simulink library "EngineSystemSubmodel"  (R2014b)
settings: Solver=ode45  StartTime=0.0  StopTime=10.0  FixedStep=1e-4  RelTol=1e-3
values from neighbouring files (symbols this model uses):
  D_turb_wheel = TC.TC_map.turb.D_wheel    [init_MVM.m]
  delta = 2    [Init8RTFLEX68D.m]    (also in Untitled2.m = fcn(p); fcn.m = zeros(size(p)))
  eta_turb_max = TC.TC_map.turb.eff_max    [init_MVM.m]
  flow_coeff_turb = [-1.585326540339;-4.823836967181;1.5853156139822]    [Init8RTFLEX68D.m]    (also in init_MVM.m = TC.TC_map.turb.flow_fit_coeff)
  fs = 0.0683    [Init8RTFLEX68D.m]    (also in NOxProcessGUI.m = varargin{2}; initHybrid.m; initMV.m; init_MVM.m = 0.0682925799315)
  genset = generators(1)    [runTempCyl4S.m]
  J_tc = TC.SAE_map_comp.inertia    [init_MVM.m]
  kai = 1.7    [Init8RTFLEX68D.m]
  Kb = 1*ones(engines,1)    [initHybrid.m]    (also in initMV.m; init_MVM.m = 1; init_ele.m = 1)
  Kd = 20*ones(engines,1)    [initHybrid.m]    (also in initMV.m; init_MVM.m = 10; init_ele.m = 20)
  Ki = 20*ones(engines,1)    [initHybrid.m]    (also in initMV.m; init_MVM.m = 10; init_ele.m = 20)
  Kp = 20*ones(engines,1)    [initHybrid.m]    (also in initMV.m; init_MVM.m = 10; init_ele.m = 20)
  Load_amp = x(4) + xRef(i)    [GetErrGensetResp.m]    (also in runsimulation.m = 0.55; runsimulationRecovery.m = InitialLoad(jj) + LoadStep(ii))
  Load_bias = x(4)    [GetErrGensetResp.m]    (also in runsimulation.m = 0.15; runsimulationRecovery.m = InitialLoad(jj))
  Load_index = 1    [GetErrGensetResp.m]    (also in runsimulation.m; runsimulationRecovery.m)
  N = x*noMol    [NOxProcessGUI.m]    (also in initHybrid.m = .1*ones(engines,1); initMV.m = .1*ones(engines,1); init_ele.m = 0.1)
  omegat0 = RPM_TC_initial/30*pi    [init_MVM.m]
  Start_time = 50    [GetErrGensetResp.m]    (also in runsimulation.m; runsimulationRecovery.m)
  T_load = 1    [GetErrGensetResp.m]    (also in runsimulation.m; runsimulationRecovery.m)
  T_ref_turb = TC.TC_map.turb.T_ref    [init_MVM.m]
  u0 = 0.2    [init_MVM.m]
  Uc_opt = TC.TC_map.turb.Uc_opt    [init_MVM.m]
  uMax = 1.5*ones(engines,1)    [initHybrid.m]    (also in initMV.m; init_MVM.m = 1.1; init_ele.m = 1.1)
  uMin = 0*ones(engines,1)    [initHybrid.m]    (also in initMV.m; init_MVM.m = 0.1; init_ele.m = 0.1)
undefined symbols (not defined in the file or in its folder): CAIPO, control, CV, cyl, eng, engSCont, omega0, rhoG0, Td, Ti, turbo, u_max, volDisp, vSCont, vSDes
undefined symbols (not defined in the file): comp_eff_map, comp_flow_map, n288_rep, npr, nsp, pr_rep, vComp
libraries: EngineSystemSubmodel x167, simulink x2
(part 3 of 5)

== system EngineSystemSubmodel/Components/EngineCylinderBlock2StrokeBusSSTune ==
  note: `
  note: `
  note: `
  note: `
  note: `
  note: `
  note: `
  uGov : Inport
  phiInj : Inport  Port=2
  cAStartNom : Inport  Port=3
  dCALiftUp : Inport  Port=4
  pTFScav : Inport  Port=5
  pTFExh : Inport  Port=6
  omega : Inport  Port=7
  tempWall : Inport  Port=8
  Bus Creator : BusCreator  Inputs=8
  Bus Creator{1..7} (7 alike) : BusCreator  Inputs=10
  Bus Selector{1..7} (7 alike) : BusSelector  OutputSignals=uGov,phiInj,CAStartNom,EVC,pTFScav,pTFExh,omegaE,tempWall
  Bus Selector{8..11,13..15} (7 alike) : BusSelector  OutputSignals=dmEmb_u,dmEmb_d,Tq,dmb
  Bus Selector16 : BusSelector  OutputSignals=pCyl,phi,V
  EngCylinder2StrokeBusSSTune1 : EngineSystemSubmodel/Components/EngCylinder2StrokeBusSSTune  cylPar=eng.cyl  cylNo=1  cyl=eng.cyl
  EngCylinder2StrokeBusSSTune2 : EngineSystemSubmodel/Components/EngCylinder2StrokeBusSSTune  cylPar=eng.cyl  cylNo=2  cyl=eng.cyl
  EngCylinder2StrokeBusSSTune3 : EngineSystemSubmodel/Components/EngCylinder2StrokeBusSSTune  cylPar=eng.cyl  cylNo=3  cyl=eng.cyl
  EngCylinder2StrokeBusSSTune4 : EngineSystemSubmodel/Components/EngCylinder2StrokeBusSSTune  cylPar=eng.cyl  cylNo=4  cyl=eng.cyl
  EngCylinder2StrokeBusSSTune5 : EngineSystemSubmodel/Components/EngCylinder2StrokeBusSSTune  cylPar=eng.cyl  cylNo=5  cyl=eng.cyl
  EngCylinder2StrokeBusSSTune6 : EngineSystemSubmodel/Components/EngCylinder2StrokeBusSSTune  cylPar=eng.cyl  cylNo=6  cyl=eng.cyl
  EngCylinder2StrokeBusSSTune7 : EngineSystemSubmodel/Components/EngCylinder2StrokeBusSSTune  cylPar=eng.cyl  cylNo=7  cyl=eng.cyl
  Sum{,1..3} (4 alike) : Sum  Inputs=+++++++
  Terminator : Terminator
  pMaxFinder : EngineSystemSubmodel/EngineOperatingParameterCalculation/pMaxFinder
  dmEmbScvg : Outport
  dmEmbExh : Outport  Port=2
  Tq : Outport  Port=3
  pMax : Outport  Port=4
  pCyl1 : Outport  Port=5
  vCyl1 : Outport  Port=6
  dmf : Outport  Port=7
  wires:
  EngCylinder2StrokeBusSSTune1/9 -> Bus Creator1/9
  [toCylinder] -> Bus Selector1/1
  pMaxFinder/1 -> pMax/1  "pMax"
  pMaxFinder/2 -> Terminator/1
  uGov/1 -> Bus Creator/1  "uGov"
  phiInj/1 -> Bus Creator/2  "phiInj"
  cAStartNom/1 -> Bus Creator/3  "CAStartNom"
  dCALiftUp/1 -> Bus Creator/4  "EVC"
  pTFScav/1 -> Bus Creator/5  "pTFScav"
  pTFExh/1 -> Bus Creator/6  "pTFExh"
  omega/1 -> Bus Creator/7  "omegaE"
  Bus Creator/1 -> [toCylinder]
  EngCylinder2StrokeBusSSTune1/1 -> pCyl1/1, Bus Creator1/1  "pCyl"
  EngCylinder2StrokeBusSSTune1/2 -> Bus Creator1/2  "phi"
  EngCylinder2StrokeBusSSTune1/3 -> Bus Creator1/3  "phiIg"
  EngCylinder2StrokeBusSSTune1/4 -> Bus Creator1/4  "dQ"
  EngCylinder2StrokeBusSSTune1/5 -> Bus Creator1/5  "dmEmb_u"
  EngCylinder2StrokeBusSSTune1/6 -> Bus Creator1/6  "dmEmb_d"
  EngCylinder2StrokeBusSSTune1/7 -> Bus Creator1/7  "Tq"
  EngCylinder2StrokeBusSSTune1/8 -> Bus Creator1/8  "dmb"
  Bus Creator1/1 -> Bus Selector16/1, Bus Selector8/1
  Bus Selector8/1 -> Sum/1  "<dmEmb_u>"
  Bus Selector9/1 -> Sum/2  "<dmEmb_u>"
  Bus Selector10/1 -> Sum/3  "<dmEmb_u>"
  Bus Selector11/1 -> Sum/4  "<dmEmb_u>"
  Bus Selector15/1 -> Sum/5  "<dmEmb_u>"
  Bus Selector14/1 -> Sum/6  "<dmEmb_u>"
  Bus Selector13/1 -> Sum/7  "<dmEmb_u>"
  Sum/1 -> dmEmbScvg/1
  Bus Selector8/2 -> Sum1/1  "<dmEmb_d>"
  Bus Selector9/2 -> Sum1/2  "<dmEmb_d>"
  Bus Selector10/2 -> Sum1/3  "<dmEmb_d>"
  Bus Selector11/2 -> Sum1/4  "<dmEmb_d>"
  Bus Selector15/2 -> Sum1/5  "<dmEmb_d>"
  Bus Selector14/2 -> Sum1/6  "<dmEmb_d>"
  Bus Selector13/2 -> Sum1/7  "<dmEmb_d>"
  Sum1/1 -> dmEmbExh/1
  Bus Selector8/3 -> Sum2/1  "<Tq>"
  Bus Selector9/3 -> Sum2/2  "<Tq>"
  Bus Selector10/3 -> Sum2/3  "<Tq>"
  Bus Selector11/3 -> Sum2/4  "<Tq>"
  Bus Selector15/3 -> Sum2/5  "<Tq>"
  Bus Selector14/3 -> Sum2/6  "<Tq>"
  Bus Selector13/3 -> Sum2/7  "<Tq>"
  Sum2/1 -> Tq/1
  Bus Selector8/4 -> Sum3/1  "<dmb>"
  Bus Selector9/4 -> Sum3/2  "<dmb>"
  Bus Selector10/4 -> Sum3/3  "<dmb>"
  Bus Selector11/4 -> Sum3/4  "<dmb>"
  Bus Selector15/4 -> Sum3/5  "<dmb>"
  Bus Selector14/4 -> Sum3/6  "<dmb>"
  Bus Selector13/4 -> Sum3/7  "<dmb>"
  Sum3/1 -> dmf/1  "dmf"
  Bus Selector16/1 -> pMaxFinder/2  "<pCyl>"
  Bus Selector16/2 -> pMaxFinder/1  "<phi>"
  Bus Selector16/3 -> vCyl1/1  "<V>"
  EngCylinder2StrokeBusSSTune1/10 -> Bus Creator1/10
  tempWall/1 -> Bus Creator/8  "tempWall"
  Bus Selector1/1 -> EngCylinder2StrokeBusSSTune1/1  "<uGov>"
  Bus Selector1/2 -> EngCylinder2StrokeBusSSTune1/2  "<phiInj>"
  Bus Selector1/3 -> EngCylinder2StrokeBusSSTune1/3  "<CAStartNom>"
  Bus Selector1/4 -> EngCylinder2StrokeBusSSTune1/4  "<EVC>"
  Bus Selector1/5 -> EngCylinder2StrokeBusSSTune1/5  "<pTFScav>"
  Bus Selector1/6 -> EngCylinder2StrokeBusSSTune1/6  "<pTFExh>"
  Bus Selector1/7 -> EngCylinder2StrokeBusSSTune1/7  "<omegaE>"
  Bus Selector1/8 -> EngCylinder2StrokeBusSSTune1/8  "<tempWall>"
  EngCylinder2StrokeBusSSTune2/9 -> Bus Creator2/9
  [toCylinder] -> Bus Selector2/1
  EngCylinder2StrokeBusSSTune2/1 -> Bus Creator2/1
  EngCylinder2StrokeBusSSTune2/2 -> Bus Creator2/2  "phi"
  EngCylinder2StrokeBusSSTune2/3 -> Bus Creator2/3  "phiIg"
  EngCylinder2StrokeBusSSTune2/4 -> Bus Creator2/4  "dQ"
  EngCylinder2StrokeBusSSTune2/5 -> Bus Creator2/5  "dmEmb_u"
  EngCylinder2StrokeBusSSTune2/6 -> Bus Creator2/6  "dmEmb_d"
  EngCylinder2StrokeBusSSTune2/7 -> Bus Creator2/7  "Tq"
  EngCylinder2StrokeBusSSTune2/8 -> Bus Creator2/8  "dmb"
  EngCylinder2StrokeBusSSTune2/10 -> Bus Creator2/10
  Bus Selector2/1 -> EngCylinder2StrokeBusSSTune2/1  "<uGov>"
  Bus Selector2/2 -> EngCylinder2StrokeBusSSTune2/2  "<phiInj>"
  Bus Selector2/3 -> EngCylinder2StrokeBusSSTune2/3  "<CAStartNom>"
  Bus Selector2/4 -> EngCylinder2StrokeBusSSTune2/4  "<EVC>"
  Bus Selector2/5 -> EngCylinder2StrokeBusSSTune2/5  "<pTFScav>"
  Bus Selector2/6 -> EngCylinder2StrokeBusSSTune2/6  "<pTFExh>"
  Bus Selector2/7 -> EngCylinder2StrokeBusSSTune2/7  "<omegaE>"
  Bus Selector2/8 -> EngCylinder2StrokeBusSSTune2/8  "<tempWall>"
  Bus Creator2/1 -> Bus Selector9/1
  EngCylinder2StrokeBusSSTune3/9 -> Bus Creator3/9
  [toCylinder] -> Bus Selector3/1
  EngCylinder2StrokeBusSSTune3/1 -> Bus Creator3/1
  EngCylinder2StrokeBusSSTune3/2 -> Bus Creator3/2  "phi"
  EngCylinder2StrokeBusSSTune3/3 -> Bus Creator3/3  "phiIg"
  EngCylinder2StrokeBusSSTune3/4 -> Bus Creator3/4  "dQ"
  EngCylinder2StrokeBusSSTune3/5 -> Bus Creator3/5  "dmEmb_u"
  EngCylinder2StrokeBusSSTune3/6 -> Bus Creator3/6  "dmEmb_d"
  EngCylinder2StrokeBusSSTune3/7 -> Bus Creator3/7  "Tq"
  EngCylinder2StrokeBusSSTune3/8 -> Bus Creator3/8  "dmb"
  EngCylinder2StrokeBusSSTune3/10 -> Bus Creator3/10
  Bus Selector3/1 -> EngCylinder2StrokeBusSSTune3/1  "<uGov>"
  Bus Selector3/2 -> EngCylinder2StrokeBusSSTune3/2  "<phiInj>"
  Bus Selector3/3 -> EngCylinder2StrokeBusSSTune3/3  "<CAStartNom>"
  Bus Selector3/4 -> EngCylinder2StrokeBusSSTune3/4  "<EVC>"
  Bus Selector3/5 -> EngCylinder2StrokeBusSSTune3/5  "<pTFScav>"
  Bus Selector3/6 -> EngCylinder2StrokeBusSSTune3/6  "<pTFExh>"
  Bus Selector3/7 -> EngCylinder2StrokeBusSSTune3/7  "<omegaE>"
  Bus Selector3/8 -> EngCylinder2StrokeBusSSTune3/8  "<tempWall>"
  Bus Creator3/1 -> Bus Selector10/1
  EngCylinder2StrokeBusSSTune4/9 -> Bus Creator4/9
  [toCylinder] -> Bus Selector4/1
  EngCylinder2StrokeBusSSTune4/1 -> Bus Creator4/1
  EngCylinder2StrokeBusSSTune4/2 -> Bus Creator4/2  "phi"
  EngCylinder2StrokeBusSSTune4/3 -> Bus Creator4/3  "phiIg"
  EngCylinder2StrokeBusSSTune4/4 -> Bus Creator4/4  "dQ"
  EngCylinder2StrokeBusSSTune4/5 -> Bus Creator4/5  "dmEmb_u"
  EngCylinder2StrokeBusSSTune4/6 -> Bus Creator4/6  "dmEmb_d"
  EngCylinder2StrokeBusSSTune4/7 -> Bus Creator4/7  "Tq"
  EngCylinder2StrokeBusSSTune4/8 -> Bus Creator4/8  "dmb"
  EngCylinder2StrokeBusSSTune4/10 -> Bus Creator4/10
  Bus Selector4/1 -> EngCylinder2StrokeBusSSTune4/1  "<uGov>"
  Bus Selector4/2 -> EngCylinder2StrokeBusSSTune4/2  "<phiInj>"
  Bus Selector4/3 -> EngCylinder2StrokeBusSSTune4/3  "<CAStartNom>"
  Bus Selector4/4 -> EngCylinder2StrokeBusSSTune4/4  "<EVC>"
  Bus Selector4/5 -> EngCylinder2StrokeBusSSTune4/5  "<pTFScav>"
  Bus Selector4/6 -> EngCylinder2StrokeBusSSTune4/6  "<pTFExh>"
  Bus Selector4/7 -> EngCylinder2StrokeBusSSTune4/7  "<omegaE>"
  Bus Selector4/8 -> EngCylinder2StrokeBusSSTune4/8  "<tempWall>"
  Bus Creator4/1 -> Bus Selector11/1
  EngCylinder2StrokeBusSSTune5/9 -> Bus Creator5/9
  [toCylinder] -> Bus Selector5/1
  EngCylinder2StrokeBusSSTune5/1 -> Bus Creator5/1
  EngCylinder2StrokeBusSSTune5/2 -> Bus Creator5/2  "phi"
  EngCylinder2StrokeBusSSTune5/3 -> Bus Creator5/3  "phiIg"
  EngCylinder2StrokeBusSSTune5/4 -> Bus Creator5/4  "dQ"
  EngCylinder2StrokeBusSSTune5/5 -> Bus Creator5/5  "dmEmb_u"
  EngCylinder2StrokeBusSSTune5/6 -> Bus Creator5/6  "dmEmb_d"
  EngCylinder2StrokeBusSSTune5/7 -> Bus Creator5/7  "Tq"
  EngCylinder2StrokeBusSSTune5/8 -> Bus Creator5/8  "dmb"
  EngCylinder2StrokeBusSSTune5/10 -> Bus Creator5/10
  Bus Selector5/1 -> EngCylinder2StrokeBusSSTune5/1  "<uGov>"
  Bus Selector5/2 -> EngCylinder2StrokeBusSSTune5/2  "<phiInj>"
  Bus Selector5/3 -> EngCylinder2StrokeBusSSTune5/3  "<CAStartNom>"
  Bus Selector5/4 -> EngCylinder2StrokeBusSSTune5/4  "<EVC>"
  Bus Selector5/5 -> EngCylinder2StrokeBusSSTune5/5  "<pTFScav>"
  Bus Selector5/6 -> EngCylinder2StrokeBusSSTune5/6  "<pTFExh>"
  Bus Selector5/7 -> EngCylinder2StrokeBusSSTune5/7  "<omegaE>"
  Bus Selector5/8 -> EngCylinder2StrokeBusSSTune5/8  "<tempWall>"
  Bus Creator5/1 -> Bus Selector15/1
  EngCylinder2StrokeBusSSTune6/9 -> Bus Creator6/9
  [toCylinder] -> Bus Selector6/1
  EngCylinder2StrokeBusSSTune6/1 -> Bus Creator6/1
  EngCylinder2StrokeBusSSTune6/2 -> Bus Creator6/2  "phi"
  EngCylinder2StrokeBusSSTune6/3 -> Bus Creator6/3  "phiIg"
  EngCylinder2StrokeBusSSTune6/4 -> Bus Creator6/4  "dQ"
  EngCylinder2StrokeBusSSTune6/5 -> Bus Creator6/5  "dmEmb_u"
  EngCylinder2StrokeBusSSTune6/6 -> Bus Creator6/6  "dmEmb_d"
  EngCylinder2StrokeBusSSTune6/7 -> Bus Creator6/7  "Tq"
  EngCylinder2StrokeBusSSTune6/8 -> Bus Creator6/8  "dmb"
  EngCylinder2StrokeBusSSTune6/10 -> Bus Creator6/10
  Bus Selector6/1 -> EngCylinder2StrokeBusSSTune6/1  "<uGov>"
  Bus Selector6/2 -> EngCylinder2StrokeBusSSTune6/2  "<phiInj>"
  Bus Selector6/3 -> EngCylinder2StrokeBusSSTune6/3  "<CAStartNom>"
  Bus Selector6/4 -> EngCylinder2StrokeBusSSTune6/4  "<EVC>"
  Bus Selector6/5 -> EngCylinder2StrokeBusSSTune6/5  "<pTFScav>"
  Bus Selector6/6 -> EngCylinder2StrokeBusSSTune6/6  "<pTFExh>"
  Bus Selector6/7 -> EngCylinder2StrokeBusSSTune6/7  "<omegaE>"
  Bus Selector6/8 -> EngCylinder2StrokeBusSSTune6/8  "<tempWall>"
  Bus Creator6/1 -> Bus Selector14/1
  EngCylinder2StrokeBusSSTune7/9 -> Bus Creator7/9
  [toCylinder] -> Bus Selector7/1
  EngCylinder2StrokeBusSSTune7/1 -> Bus Creator7/1
  EngCylinder2StrokeBusSSTune7/2 -> Bus Creator7/2  "phi"
  EngCylinder2StrokeBusSSTune7/3 -> Bus Creator7/3  "phiIg"
  EngCylinder2StrokeBusSSTune7/4 -> Bus Creator7/4  "dQ"
  EngCylinder2StrokeBusSSTune7/5 -> Bus Creator7/5  "dmEmb_u"
  EngCylinder2StrokeBusSSTune7/6 -> Bus Creator7/6  "dmEmb_d"
  EngCylinder2StrokeBusSSTune7/7 -> Bus Creator7/7  "Tq"
  EngCylinder2StrokeBusSSTune7/8 -> Bus Creator7/8  "dmb"
  EngCylinder2StrokeBusSSTune7/10 -> Bus Creator7/10
  Bus Selector7/1 -> EngCylinder2StrokeBusSSTune7/1  "<uGov>"
  Bus Selector7/2 -> EngCylinder2StrokeBusSSTune7/2  "<phiInj>"
  Bus Selector7/3 -> EngCylinder2StrokeBusSSTune7/3  "<CAStartNom>"
  Bus Selector7/4 -> EngCylinder2StrokeBusSSTune7/4  "<EVC>"
  Bus Selector7/5 -> EngCylinder2StrokeBusSSTune7/5  "<pTFScav>"
  Bus Selector7/6 -> EngCylinder2StrokeBusSSTune7/6  "<pTFExh>"
  Bus Selector7/7 -> EngCylinder2StrokeBusSSTune7/7  "<omegaE>"
  Bus Selector7/8 -> EngCylinder2StrokeBusSSTune7/8  "<tempWall>"
  Bus Creator7/1 -> Bus Selector13/1

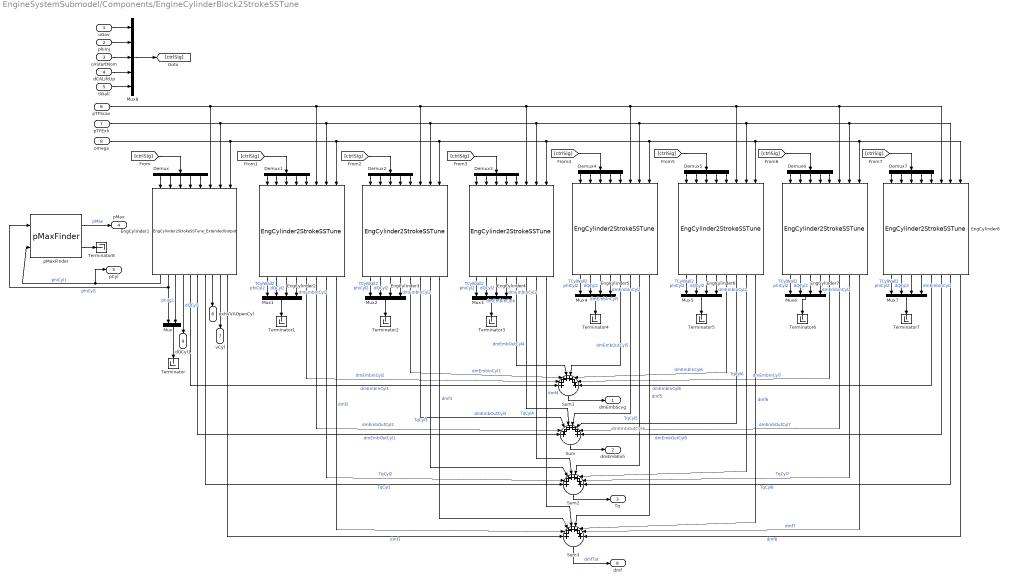
== system EngineSystemSubmodel/Components/EngineCylinderBlock2StrokeSSTune ==
  note: dmEmbOutCyl6
  uGov : Inport
  phiInj : Inport  Port=2
  cAStartNom : Inport  Port=3
  dCALiftUp : Inport  Port=4
  tWall : Inport  Port=5
  pTFScav : Inport  Port=6
  pTFExh : Inport  Port=7
  omega : Inport  Port=8
  Demux{,1..7} (8 alike) : Demux  Outputs=5
  EngCylinder1 : EngineSystemSubmodel/Components/EngCylinder2StrokeSSTune_ExtendedOutput  cylPar=eng.cyl  cylNo=1  cyl=eng.cyl
  EngCylinder2 : EngineSystemSubmodel/Components/EngCylinder2StrokeSSTune  cylPar=eng.cyl  cylNo=2  cyl=eng.cyl
  EngCylinder3 : EngineSystemSubmodel/Components/EngCylinder2StrokeSSTune  cylPar=eng.cyl  cylNo=3  cyl=eng.cyl
  EngCylinder4 : EngineSystemSubmodel/Components/EngCylinder2StrokeSSTune  cylPar=eng.cyl  cylNo=4  cyl=eng.cyl
  EngCylinder5 : EngineSystemSubmodel/Components/EngCylinder2StrokeSSTune  cylPar=eng.cyl  cylNo=5  cyl=eng.cyl
  EngCylinder6 : EngineSystemSubmodel/Components/EngCylinder2StrokeSSTune  cylPar=eng.cyl  cylNo=6  cyl=eng.cyl
  EngCylinder7 : EngineSystemSubmodel/Components/EngCylinder2StrokeSSTune  cylPar=eng.cyl  cylNo=7  cyl=eng.cyl
  EngCylinder8 : EngineSystemSubmodel/Components/EngCylinder2StrokeSSTune  cylPar=eng.cyl  cylNo=8  cyl=eng.cyl
  Mux : Mux  Inputs=2
  Mux{1..7} (7 alike) : Mux
  Mux8 : Mux  Inputs=5
  Sum{,1..3} (4 alike) : Sum  Inputs=++++++++
  Terminator{,1..8} (9 alike) : Terminator
  pMaxFinder : EngineSystemSubmodel/EngineOperatingParameterCalculation/pMaxFinder
  dmEmbScvg : Outport
  dmEmbExh : Outport  Port=2
  Tq : Outport  Port=3
  pMax : Outport  Port=4
  pCyl : Outport  Port=5
  exhVVAOpenCyl : Outport  Port=6
  vCyl : Outport  Port=7
  dmf : Outport  Port=8
  dQCyl1 : Outport  Port=9
  wires:
  EngCylinder2/4 -> Mux1/4  "dmEmbInCyl2"
  Demux1/4 -> EngCylinder2/4
  Demux1/3 -> EngCylinder2/3
  Demux1/2 -> EngCylinder2/2
  Demux1/1 -> EngCylinder2/1
  [ctrlSig] -> Demux1/1
  Demux/4 -> EngCylinder1/4
  Demux/3 -> EngCylinder1/3
  Demux/2 -> EngCylinder1/2
  Demux/1 -> EngCylinder1/1
  [ctrlSig] -> Demux/1
  Mux8/1 -> [ctrlSig]
  dCALiftUp/1 -> Mux8/4
  cAStartNom/1 -> Mux8/3
  phiInj/1 -> Mux8/2
  uGov/1 -> Mux8/1
  Sum3/1 -> dmf/1  "dmfTot"
  EngCylinder8/8 -> Sum3/8  "dmf8"
  EngCylinder7/8 -> Sum3/7  "dmf7"
  EngCylinder6/8 -> Sum3/6  "dmf6"
  EngCylinder5/8 -> Sum3/5  "dmf5"
  EngCylinder4/8 -> Sum3/4  "dmf4"
  EngCylinder3/8 -> Sum3/3  "dmf3"
  EngCylinder2/8 -> Sum3/2  "dmf2"
  EngCylinder1/10 -> Sum3/1  "dmf1"
  EngCylinder1/9 -> vCyl/1
  EngCylinder1/8 -> exhVVAOpenCyl/1
  EngCylinder1/1 -> pMaxFinder/2, pCyl/1  "phiCyl1"
  pMaxFinder/2 -> Terminator8/1
  pMaxFinder/1 -> pMax/1  "pMax"
  Sum/1 -> dmEmbExh/1
  Sum1/1 -> dmEmbScvg/1
  Sum2/1 -> Tq/1
  EngCylinder8/5 -> Sum1/8  "dmEmbInCyl8"
  EngCylinder1/7 -> Sum2/1  "TqCyl1"
  EngCylinder2/1 -> Mux1/1  "phiCyl2"
  Mux1/1 -> Terminator1/1
  EngCylinder1/3 -> Mux/2  "phiIg1"
  EngCylinder1/4 -> dQCyl1/1  "dQCyl1"
  EngCylinder2/3 -> Mux1/3  "dQCyl2"
  EngCylinder1/2 -> pMaxFinder/1, Mux/1  "phiCyl1"
  EngCylinder2/2 -> Mux1/2  "TCylWall2"
  Mux/1 -> Terminator/1
  EngCylinder5/6 -> Sum/5  "dmEmbOutCyl5"
  EngCylinder6/6 -> Sum/6
  EngCylinder2/6 -> Sum/2  "dmEmbOutCyl2"
  EngCylinder7/5 -> Sum1/7  "dmEmbInCyl7"
  EngCylinder1/6 -> Sum/1  "dmEmbOutCyl1"
  EngCylinder3/6 -> Sum/3  "dmEmbOutCyl3"
  EngCylinder4/6 -> Sum/4  "dmEmbOutCyl4"
  EngCylinder5/5 -> Sum1/5  "dmEmbInCyl5"
  EngCylinder6/5 -> Sum1/6  "dmEmbInCyl6"
  EngCylinder4/5 -> Sum1/4  "dmEmbInCyl4"
  EngCylinder3/5 -> Sum1/3  "dmEmbInCyl3"
  EngCylinder2/5 -> Sum1/2  "dmEmbInCyl2"
  EngCylinder1/5 -> Sum1/1  "dmEmbInCyl1"
  EngCylinder5/7 -> Sum2/5  "TqCyl5"
  EngCylinder4/7 -> Sum2/4  "TqCyl4"
  EngCylinder3/7 -> Sum2/3  "TqCyl3"
  EngCylinder6/7 -> Sum2/6  "TqCyl6"
  EngCylinder8/7 -> Sum2/8  "TqCyl8"
  EngCylinder7/7 -> Sum2/7  "TqCyl7"
  EngCylinder2/7 -> Sum2/2  "TqCyl2"
  EngCylinder7/6 -> Sum/7  "dmEmbOutCyl7"
  EngCylinder8/6 -> Sum/8  "dmEmbOutCyl8"
  tWall/1 -> Mux8/5
  Demux/5 -> EngCylinder1/5
  Demux1/5 -> EngCylinder2/5
  EngCylinder3/4 -> Mux2/4  "dmEmbInCyl2"
  Demux2/4 -> EngCylinder3/4
  Demux2/3 -> EngCylinder3/3
  Demux2/2 -> EngCylinder3/2
  Demux2/1 -> EngCylinder3/1
  [ctrlSig] -> Demux2/1
  EngCylinder3/1 -> Mux2/1  "phiCyl2"
  Mux2/1 -> Terminator2/1
  EngCylinder3/3 -> Mux2/3  "dQCyl2"
  EngCylinder3/2 -> Mux2/2  "TCylWall2"
  Demux2/5 -> EngCylinder3/5
  EngCylinder4/4 -> Mux3/4  "dmEmbInCyl2"
  Demux3/4 -> EngCylinder4/4
  Demux3/3 -> EngCylinder4/3
  Demux3/2 -> EngCylinder4/2
  Demux3/1 -> EngCylinder4/1
  [ctrlSig] -> Demux3/1
  EngCylinder4/1 -> Mux3/1  "phiCyl2"
  Mux3/1 -> Terminator3/1
  EngCylinder4/3 -> Mux3/3  "dQCyl2"
  EngCylinder4/2 -> Mux3/2  "TCylWall2"
  Demux3/5 -> EngCylinder4/5
  EngCylinder5/4 -> Mux4/4  "dmEmbInCyl2"
  Demux4/4 -> EngCylinder5/4
  Demux4/3 -> EngCylinder5/3
  Demux4/2 -> EngCylinder5/2
  Demux4/1 -> EngCylinder5/1
  [ctrlSig] -> Demux4/1
  EngCylinder5/1 -> Mux4/1  "phiCyl2"
  Mux4/1 -> Terminator4/1
  EngCylinder5/3 -> Mux4/3  "dQCyl2"
  EngCylinder5/2 -> Mux4/2  "TCylWall2"
  Demux4/5 -> EngCylinder5/5
  EngCylinder6/4 -> Mux5/4  "dmEmbInCyl2"
  Demux5/4 -> EngCylinder6/4
  Demux5/3 -> EngCylinder6/3
  Demux5/2 -> EngCylinder6/2
  Demux5/1 -> EngCylinder6/1
  [ctrlSig] -> Demux5/1
  EngCylinder6/1 -> Mux5/1  "phiCyl2"
  Mux5/1 -> Terminator5/1
  EngCylinder6/3 -> Mux5/3  "dQCyl2"
  EngCylinder6/2 -> Mux5/2  "TCylWall2"
  Demux5/5 -> EngCylinder6/5
  EngCylinder7/4 -> Mux6/4  "dmEmbInCyl2"
  Demux6/4 -> EngCylinder7/4
  Demux6/3 -> EngCylinder7/3
  Demux6/2 -> EngCylinder7/2
  Demux6/1 -> EngCylinder7/1
  [ctrlSig] -> Demux6/1
  omega/1 -> EngCylinder1/8, EngCylinder2/8, EngCylinder5/8, EngCylinder8/8, EngCylinder7/8, EngCylinder6/8, EngCylinder4/8, EngCylinder3/8
  pTFExh/1 -> EngCylinder1/7, EngCylinder2/7, EngCylinder5/7, EngCylinder7/7, EngCylinder8/7, EngCylinder6/7, EngCylinder4/7, EngCylinder3/7
  EngCylinder7/1 -> Mux6/1  "phiCyl2"
  Mux6/1 -> Terminator6/1
  EngCylinder7/3 -> Mux6/3  "dQCyl2"
  EngCylinder7/2 -> Mux6/2  "TCylWall2"
  pTFScav/1 -> EngCylinder1/6, EngCylinder2/6, EngCylinder5/6, EngCylinder7/6, EngCylinder8/6, EngCylinder6/6, EngCylinder4/6, EngCylinder3/6
  Demux6/5 -> EngCylinder7/5
  EngCylinder8/4 -> Mux7/4  "dmEmbInCyl2"
  Demux7/4 -> EngCylinder8/4
  Demux7/3 -> EngCylinder8/3
  Demux7/2 -> EngCylinder8/2
  Demux7/1 -> EngCylinder8/1
  [ctrlSig] -> Demux7/1
  EngCylinder8/1 -> Mux7/1  "phiCyl2"
  Mux7/1 -> Terminator7/1
  EngCylinder8/3 -> Mux7/3  "dQCyl2"
  Demux7/5 -> EngCylinder8/5
  EngCylinder8/2 -> Mux7/2  "TCylWall2"

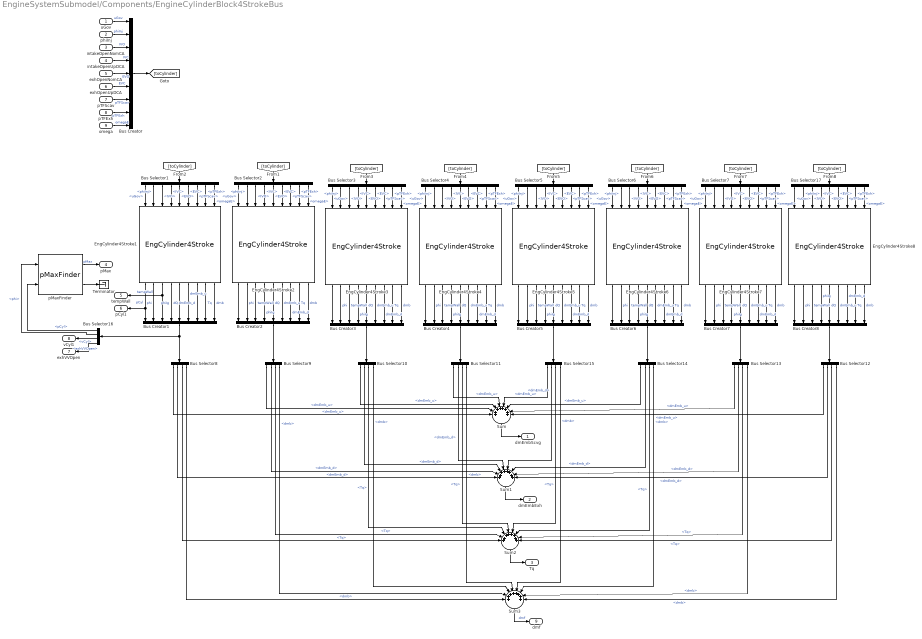
== system EngineSystemSubmodel/Components/EngineCylinderBlock4StrokeBus ==
  uGov : Inport
  phiInj : Inport  Port=2
  intakeOpenNomCA : Inport  Port=3
  intakeOpenUpDCA : Inport  Port=4
  exhOpenNomCA : Inport  Port=5
  exhOpenUpDCA : Inport  Port=6
  pTFScav : Inport  Port=7
  pTFExh : Inport  Port=8
  omega : Inport  Port=9
  Bus Creator{,1..8} (9 alike) : BusCreator  Inputs=9
  Bus Selector{1..7,17} (8 alike) : BusSelector  OutputSignals=uGov,phiInj,IVO,IVC,EVO,EVC,pTFScav,pTFExh,omegaE
  Bus Selector{8..15} (8 alike) : BusSelector  OutputSignals=dmEmb_u,dmEmb_d,Tq,dmb
  Bus Selector16 : BusSelector  OutputSignals=pCyl,phi,vCyl,exhVVOpen
  EngCylinder4Stroke{1..8} (8 alike) : EngineSystemSubmodel/Components/EngCylinder4Stroke  cyl=eng.cyl  cylNo=1
  Sum{,1..3} (4 alike) : Sum  Inputs=++++++++
  Terminator : Terminator
  pMaxFinder : EngineSystemSubmodel/EngineOperatingParameterCalculation/pMaxFinder
  dmEmbScvg : Outport
  dmEmbExh : Outport  Port=2
  Tq : Outport  Port=3
  pMax : Outport  Port=4
  tempWall : Outport  Port=5
  pCyl1 : Outport  Port=6
  exhVVOpen : Outport  Port=7
  vCyl1 : Outport  Port=8
  dmf : Outport  Port=9
  wires:
  Bus Selector16/4 -> exhVVOpen/1  "<exhVVOpen>"
  Bus Selector16/3 -> vCyl1/1  "<vCyl>"
  EngCylinder4Stroke1/3 -> tempWall/1, Bus Creator1/3  "tempWall"
  Bus Selector16/2 -> pMaxFinder/1  "<phi>"
  Bus Selector16/1 -> pMaxFinder/2  "<pCyl>"
  Sum3/1 -> dmf/1  "dmf"
  Bus Selector12/4 -> Sum3/8  "<dmb>"
  Bus Selector13/4 -> Sum3/7  "<dmb>"
  Bus Selector14/4 -> Sum3/6  "<dmb>"
  Bus Selector15/4 -> Sum3/5  "<dmb>"
  Bus Selector11/4 -> Sum3/4  "<dmb>"
  Bus Selector10/4 -> Sum3/3  "<dmb>"
  Bus Selector9/4 -> Sum3/2  "<dmb>"
  Bus Selector8/4 -> Sum3/1  "<dmb>"
  Sum2/1 -> Tq/1
  Bus Selector12/3 -> Sum2/8  "<Tq>"
  Bus Selector13/3 -> Sum2/7  "<Tq>"
  Bus Selector14/3 -> Sum2/6  "<Tq>"
  Bus Selector15/3 -> Sum2/5  "<Tq>"
  Bus Selector11/3 -> Sum2/4  "<Tq>"
  Bus Selector10/3 -> Sum2/3  "<Tq>"
  Bus Selector9/3 -> Sum2/2  "<Tq>"
  Bus Selector8/3 -> Sum2/1  "<Tq>"
  Sum1/1 -> dmEmbExh/1
  Bus Selector12/2 -> Sum1/8  "<dmEmb_d>"
  Bus Selector13/2 -> Sum1/7  "<dmEmb_d>"
  Bus Selector14/2 -> Sum1/6  "<dmEmb_d>"
  Bus Selector15/2 -> Sum1/5  "<dmEmb_d>"
  Bus Selector11/2 -> Sum1/4  "<dmEmb_d>"
  Bus Selector10/2 -> Sum1/3  "<dmEmb_d>"
  Bus Selector9/2 -> Sum1/2  "<dmEmb_d>"
  Bus Selector8/2 -> Sum1/1  "<dmEmb_d>"
  Sum/1 -> dmEmbScvg/1
  Bus Selector12/1 -> Sum/8  "<dmEmb_u>"
  Bus Selector13/1 -> Sum/7  "<dmEmb_u>"
  Bus Selector14/1 -> Sum/6  "<dmEmb_u>"
  Bus Selector15/1 -> Sum/5  "<dmEmb_u>"
  Bus Selector11/1 -> Sum/4  "<dmEmb_u>"
  Bus Selector10/1 -> Sum/3  "<dmEmb_u>"
  Bus Selector9/1 -> Sum/2  "<dmEmb_u>"
  Bus Selector8/1 -> Sum/1  "<dmEmb_u>"
  Bus Creator1/1 -> Bus Selector16/1, Bus Selector8/1
  EngCylinder4Stroke1/9 -> Bus Creator1/9  "dmb"
  EngCylinder4Stroke1/8 -> Bus Creator1/8  "Tq"
  EngCylinder4Stroke1/7 -> Bus Creator1/7  "dmEmb_d"
  EngCylinder4Stroke1/6 -> Bus Creator1/6  "dmEmb_u"
  EngCylinder4Stroke1/5 -> Bus Creator1/5  "dQ"
  EngCylinder4Stroke1/4 -> Bus Creator1/4  "phiIg"
  EngCylinder4Stroke1/2 -> Bus Creator1/2  "phi"
  EngCylinder4Stroke1/1 -> pCyl1/1, Bus Creator1/1  "pCyl"
  Bus Creator/1 -> [toCylinder]
  omega/1 -> Bus Creator/9  "omegaE"
  pTFExh/1 -> Bus Creator/8  "pTFExh"
  pTFScav/1 -> Bus Creator/7  "pTFScav"
  exhOpenUpDCA/1 -> Bus Creator/6  "EVC"
  exhOpenNomCA/1 -> Bus Creator/5  "EVO"
  phiInj/1 -> Bus Creator/2  "phiInj"
  uGov/1 -> Bus Creator/1  "uGov"
  pMaxFinder/2 -> Terminator/1
  pMaxFinder/1 -> pMax/1  "pMax"
  [toCylinder] -> Bus Selector1/1
  intakeOpenNomCA/1 -> Bus Creator/3  "IVO"
  intakeOpenUpDCA/1 -> Bus Creator/4  "IVC"
  Bus Selector1/1 -> EngCylinder4Stroke1/1  "<uGov>"
  Bus Selector1/2 -> EngCylinder4Stroke1/2  "<phiInj>"
  Bus Selector1/3 -> EngCylinder4Stroke1/3  "<IVO>"
  Bus Selector1/4 -> EngCylinder4Stroke1/4  "<IVC>"
  Bus Selector1/5 -> EngCylinder4Stroke1/5  "<EVO>"
  Bus Selector1/6 -> EngCylinder4Stroke1/6  "<EVC>"
  Bus Selector1/7 -> EngCylinder4Stroke1/7  "<pTFScav>"
  Bus Selector1/8 -> EngCylinder4Stroke1/8  "<pTFExh>"
  Bus Selector1/9 -> EngCylinder4Stroke1/9  "<omegaE>"
  EngCylinder4Stroke2/3 -> Bus Creator2/3  "tempWall"
  Bus Creator2/1 -> Bus Selector9/1
  EngCylinder4Stroke2/9 -> Bus Creator2/9  "dmb"
  EngCylinder4Stroke2/8 -> Bus Creator2/8  "Tq"
  EngCylinder4Stroke2/7 -> Bus Creator2/7  "dmEmb_d"
  EngCylinder4Stroke2/6 -> Bus Creator2/6  "dmEmb_u"
  EngCylinder4Stroke2/5 -> Bus Creator2/5  "dQ"
  EngCylinder4Stroke2/4 -> Bus Creator2/4  "phiIg"
  EngCylinder4Stroke2/2 -> Bus Creator2/2  "phi"
  EngCylinder4Stroke2/1 -> Bus Creator2/1
  [toCylinder] -> Bus Selector2/1
  Bus Selector2/1 -> EngCylinder4Stroke2/1  "<uGov>"
  Bus Selector2/2 -> EngCylinder4Stroke2/2  "<phiInj>"
  Bus Selector2/3 -> EngCylinder4Stroke2/3  "<IVO>"
  Bus Selector2/4 -> EngCylinder4Stroke2/4  "<IVC>"
  Bus Selector2/5 -> EngCylinder4Stroke2/5  "<EVO>"
  Bus Selector2/6 -> EngCylinder4Stroke2/6  "<EVC>"
  Bus Selector2/7 -> EngCylinder4Stroke2/7  "<pTFScav>"
  Bus Selector2/8 -> EngCylinder4Stroke2/8  "<pTFExh>"
  Bus Selector2/9 -> EngCylinder4Stroke2/9  "<omegaE>"
  EngCylinder4Stroke3/3 -> Bus Creator3/3  "tempWall"
  Bus Creator3/1 -> Bus Selector10/1
  EngCylinder4Stroke3/9 -> Bus Creator3/9  "dmb"
  EngCylinder4Stroke3/8 -> Bus Creator3/8  "Tq"
  EngCylinder4Stroke3/7 -> Bus Creator3/7  "dmEmb_d"
  EngCylinder4Stroke3/6 -> Bus Creator3/6  "dmEmb_u"
  EngCylinder4Stroke3/5 -> Bus Creator3/5  "dQ"
  EngCylinder4Stroke3/4 -> Bus Creator3/4  "phiIg"
  EngCylinder4Stroke3/2 -> Bus Creator3/2  "phi"
  EngCylinder4Stroke3/1 -> Bus Creator3/1
  [toCylinder] -> Bus Selector3/1
  Bus Selector3/1 -> EngCylinder4Stroke3/1  "<uGov>"
  Bus Selector3/2 -> EngCylinder4Stroke3/2  "<phiInj>"
  Bus Selector3/3 -> EngCylinder4Stroke3/3  "<IVO>"
  Bus Selector3/4 -> EngCylinder4Stroke3/4  "<IVC>"
  Bus Selector3/5 -> EngCylinder4Stroke3/5  "<EVO>"
  Bus Selector3/6 -> EngCylinder4Stroke3/6  "<EVC>"
  Bus Selector3/7 -> EngCylinder4Stroke3/7  "<pTFScav>"
  Bus Selector3/8 -> EngCylinder4Stroke3/8  "<pTFExh>"
  Bus Selector3/9 -> EngCylinder4Stroke3/9  "<omegaE>"
  EngCylinder4Stroke4/3 -> Bus Creator4/3  "tempWall"
  Bus Creator4/1 -> Bus Selector11/1
  EngCylinder4Stroke4/9 -> Bus Creator4/9  "dmb"
  EngCylinder4Stroke4/8 -> Bus Creator4/8  "Tq"
  EngCylinder4Stroke4/7 -> Bus Creator4/7  "dmEmb_d"
  EngCylinder4Stroke4/6 -> Bus Creator4/6  "dmEmb_u"
  EngCylinder4Stroke4/5 -> Bus Creator4/5  "dQ"
  EngCylinder4Stroke4/4 -> Bus Creator4/4  "phiIg"
  EngCylinder4Stroke4/2 -> Bus Creator4/2  "phi"
  EngCylinder4Stroke4/1 -> Bus Creator4/1
  [toCylinder] -> Bus Selector4/1
  Bus Selector4/1 -> EngCylinder4Stroke4/1  "<uGov>"
  Bus Selector4/2 -> EngCylinder4Stroke4/2  "<phiInj>"
  Bus Selector4/3 -> EngCylinder4Stroke4/3  "<IVO>"
  Bus Selector4/4 -> EngCylinder4Stroke4/4  "<IVC>"
  Bus Selector4/5 -> EngCylinder4Stroke4/5  "<EVO>"
  Bus Selector4/6 -> EngCylinder4Stroke4/6  "<EVC>"
  Bus Selector4/7 -> EngCylinder4Stroke4/7  "<pTFScav>"
  Bus Selector4/8 -> EngCylinder4Stroke4/8  "<pTFExh>"
  Bus Selector4/9 -> EngCylinder4Stroke4/9  "<omegaE>"
  EngCylinder4Stroke5/3 -> Bus Creator5/3  "tempWall"
  Bus Creator5/1 -> Bus Selector15/1
  EngCylinder4Stroke5/9 -> Bus Creator5/9  "dmb"
  EngCylinder4Stroke5/8 -> Bus Creator5/8  "Tq"
  EngCylinder4Stroke5/7 -> Bus Creator5/7  "dmEmb_d"
  EngCylinder4Stroke5/6 -> Bus Creator5/6  "dmEmb_u"
  EngCylinder4Stroke5/5 -> Bus Creator5/5  "dQ"
  EngCylinder4Stroke5/4 -> Bus Creator5/4  "phiIg"
  EngCylinder4Stroke5/2 -> Bus Creator5/2  "phi"
  EngCylinder4Stroke5/1 -> Bus Creator5/1
  [toCylinder] -> Bus Selector5/1
  Bus Selector5/1 -> EngCylinder4Stroke5/1  "<uGov>"
  Bus Selector5/2 -> EngCylinder4Stroke5/2  "<phiInj>"
  Bus Selector5/3 -> EngCylinder4Stroke5/3  "<IVO>"
  Bus Selector5/4 -> EngCylinder4Stroke5/4  "<IVC>"
  Bus Selector5/5 -> EngCylinder4Stroke5/5  "<EVO>"
  Bus Selector5/6 -> EngCylinder4Stroke5/6  "<EVC>"
  Bus Selector5/7 -> EngCylinder4Stroke5/7  "<pTFScav>"
  Bus Selector5/8 -> EngCylinder4Stroke5/8  "<pTFExh>"
  Bus Selector5/9 -> EngCylinder4Stroke5/9  "<omegaE>"
  EngCylinder4Stroke6/3 -> Bus Creator6/3  "tempWall"
  Bus Creator6/1 -> Bus Selector14/1
  EngCylinder4Stroke6/9 -> Bus Creator6/9  "dmb"
  EngCylinder4Stroke6/8 -> Bus Creator6/8  "Tq"
  EngCylinder4Stroke6/7 -> Bus Creator6/7  "dmEmb_d"
  EngCylinder4Stroke6/6 -> Bus Creator6/6  "dmEmb_u"
  EngCylinder4Stroke6/5 -> Bus Creator6/5  "dQ"
  EngCylinder4Stroke6/4 -> Bus Creator6/4  "phiIg"
  EngCylinder4Stroke6/2 -> Bus Creator6/2  "phi"
  EngCylinder4Stroke6/1 -> Bus Creator6/1
  [toCylinder] -> Bus Selector6/1
  Bus Selector6/1 -> EngCylinder4Stroke6/1  "<uGov>"
  Bus Selector6/2 -> EngCylinder4Stroke6/2  "<phiInj>"
  Bus Selector6/3 -> EngCylinder4Stroke6/3  "<IVO>"
  Bus Selector6/4 -> EngCylinder4Stroke6/4  "<IVC>"
  Bus Selector6/5 -> EngCylinder4Stroke6/5  "<EVO>"
  Bus Selector6/6 -> EngCylinder4Stroke6/6  "<EVC>"
  Bus Selector6/7 -> EngCylinder4Stroke6/7  "<pTFScav>"
  Bus Selector6/8 -> EngCylinder4Stroke6/8  "<pTFExh>"
  Bus Selector6/9 -> EngCylinder4Stroke6/9  "<omegaE>"
  EngCylinder4Stroke7/3 -> Bus Creator7/3  "tempWall"
  Bus Creator7/1 -> Bus Selector13/1
  EngCylinder4Stroke7/9 -> Bus Creator7/9  "dmb"
  EngCylinder4Stroke7/8 -> Bus Creator7/8  "Tq"
  EngCylinder4Stroke7/7 -> Bus Creator7/7  "dmEmb_d"
  EngCylinder4Stroke7/6 -> Bus Creator7/6  "dmEmb_u"
  EngCylinder4Stroke7/5 -> Bus Creator7/5  "dQ"
  EngCylinder4Stroke7/4 -> Bus Creator7/4  "phiIg"
  EngCylinder4Stroke7/2 -> Bus Creator7/2  "phi"
  EngCylinder4Stroke7/1 -> Bus Creator7/1
  [toCylinder] -> Bus Selector7/1
  Bus Selector7/1 -> EngCylinder4Stroke7/1  "<uGov>"
  Bus Selector7/2 -> EngCylinder4Stroke7/2  "<phiInj>"
  Bus Selector7/3 -> EngCylinder4Stroke7/3  "<IVO>"
  Bus Selector7/4 -> EngCylinder4Stroke7/4  "<IVC>"
  Bus Selector7/5 -> EngCylinder4Stroke7/5  "<EVO>"
  Bus Selector7/6 -> EngCylinder4Stroke7/6  "<EVC>"
  Bus Selector7/7 -> EngCylinder4Stroke7/7  "<pTFScav>"
  Bus Selector7/8 -> EngCylinder4Stroke7/8  "<pTFExh>"
  Bus Selector7/9 -> EngCylinder4Stroke7/9  "<omegaE>"
  EngCylinder4Stroke8/3 -> Bus Creator8/3  "tempWall"
  Bus Creator8/1 -> Bus Selector12/1
  EngCylinder4Stroke8/9 -> Bus Creator8/9  "dmb"
  EngCylinder4Stroke8/8 -> Bus Creator8/8  "Tq"
  EngCylinder4Stroke8/7 -> Bus Creator8/7  "dmEmb_d"
  EngCylinder4Stroke8/6 -> Bus Creator8/6  "dmEmb_u"
  EngCylinder4Stroke8/5 -> Bus Creator8/5  "dQ"
  EngCylinder4Stroke8/4 -> Bus Creator8/4  "phiIg"
  EngCylinder4Stroke8/2 -> Bus Creator8/2  "phi"
  EngCylinder4Stroke8/1 -> Bus Creator8/1
  [toCylinder] -> Bus Selector17/1
  Bus Selector17/1 -> EngCylinder4Stroke8/1  "<uGov>"
  Bus Selector17/2 -> EngCylinder4Stroke8/2  "<phiInj>"
  Bus Selector17/3 -> EngCylinder4Stroke8/3  "<IVO>"
  Bus Selector17/4 -> EngCylinder4Stroke8/4  "<IVC>"
  Bus Selector17/5 -> EngCylinder4Stroke8/5  "<EVO>"
  Bus Selector17/6 -> EngCylinder4Stroke8/6  "<EVC>"
  Bus Selector17/7 -> EngCylinder4Stroke8/7  "<pTFScav>"
  Bus Selector17/8 -> EngCylinder4Stroke8/8  "<pTFExh>"
  Bus Selector17/9 -> EngCylinder4Stroke8/9  "<omegaE>"

== system EngineSystemSubmodel/Components/ExhValve ==
  phi : Inport
  cAStartNom : Inport  Port=2
  dCALiftUp : Inport  Port=3
  pTF_u : Inport  Port=4
  pTF_d : Inport  Port=5
  Demux : Demux  Outputs=3
  Demux1 : Demux  Outputs=3
  IdealNozzle : EngineSystemSubmodel/Flow Restriction/IdealNozzle
  S-Function : S-Function  FunctionName=GetVVLift  Parameters=eng.nStroke,cyl.exhVVDim.liftMax,cyl.exhVVProf.cAStartRef,cyl.exhVVProf.dCALiftUp,cyl.exhVVProf.dCALiftDown,cyl.exhVVProf.dCALiftTopRef,cyl.exhVVProf.cAVVUpRef,cyl.exhVVProf.cAVVDownRef,cyl.exhVVProf.liftUpRef,cyl.exhVVProf.liftDownRef  EnableBusSupport=off
  S-Function1 : S-Function  FunctionName=GetExhVVArea  Parameters=cyl.exhVVDim.Dv,cyl.exhVVDim.beta,cyl.exhVVDim.w,cyl.exhVVDim.Dp,cyl.exhVVDim.Ds,coeffCdCorrP,coeffCdCorrQ,coeffCdCorrPR  EnableBusSupport=off  mask{coeffCdCorrP=[0.5329;-0.2047;0.04292], coeffCdCorrQ=[0.5359;-0.2962;0.06275], coeffCdCorrPR=[-0.006345;0.09503;0.8117]}
      mask prompts: coeffCdCorrP "Produt coefficient for discharge coefficient for lift ratio"; coeffCdCorrQ "Quotient coefficient for discharge coefficient for lift ratio"; coeffCdCorrPR "Coefficient for discharge coefficient for pressure ratio"
  Terminator{,1..3} (4 alike) : Terminator
  dmEmb_u : Outport
  dmEmb_d : Outport  Port=2
  aOpen : Outport  Port=3
  Cd : Outport  Port=4
  wires:
  S-Function/1 -> S-Function1/1  "ExhVVlift"
  pTF_d/1 -> Demux1/1, IdealNozzle/3
  pTF_u/1 -> Demux/1, IdealNozzle/2
  IdealNozzle/2 -> dmEmb_d/1
  IdealNozzle/1 -> dmEmb_u/1
  phi/1 -> S-Function/1
  cAStartNom/1 -> S-Function/2
  dCALiftUp/1 -> S-Function/3
  S-Function1/3 -> IdealNozzle/1  "aEff"
  S-Function1/1 -> aOpen/1
  S-Function1/2 -> Cd/1
  Demux/1 -> S-Function1/2  "pIn"
  Demux1/1 -> S-Function1/3  "pOut"
  Demux/2 -> Terminator/1
  Demux/3 -> Terminator1/1
  Demux1/2 -> Terminator2/1
  Demux1/3 -> Terminator3/1

== system EngineSystemSubmodel/Components/ExhValveBus ==
  phi : Inport
  cAStartNom : Inport  Port=2
  dCALiftUp : Inport  Port=3
  pTF_u : Inport  Port=4
  pTF_d : Inport  Port=5
  Bus Selector : BusSelector  OutputSignals=p
  Bus Selector1 : BusSelector  OutputSignals=p
  IdealNozzleBus : EngineSystemSubmodel/Flow Restriction/IdealNozzleBus
  S-Function : S-Function  FunctionName=GetVVLift  Parameters=eng.nStroke,cyl.exhVVDim.liftMax,cyl.exhVVProf.cAStartRef,cyl.exhVVProf.dCALiftUp,cyl.exhVVProf.dCALiftDown,cyl.exhVVProf.dCALiftTopRef,cyl.exhVVProf.cAVVUpRef,cyl.exhVVProf.cAVVDownRef,cyl.exhVVProf.liftUpRef,cyl.exhVVProf.liftDownRef  EnableBusSupport=off
  S-Function1 : S-Function  FunctionName=GetExhVVArea  Parameters=cyl.exhVVDim.Dv,cyl.exhVVDim.beta,cyl.exhVVDim.w,cyl.exhVVDim.Dp,cyl.exhVVDim.Ds,coeffCdCorrP,coeffCdCorrQ,coeffCdCorrPR  EnableBusSupport=off  mask{coeffCdCorrP=[0.5329;-0.2047;0.04292], coeffCdCorrQ=[0.5359;-0.2962;0.06275], coeffCdCorrPR=[-0.006345;0.09503;0.8117]}
      mask prompts: coeffCdCorrP "Produt coefficient for discharge coefficient for lift ratio"; coeffCdCorrQ "Quotient coefficient for discharge coefficient for lift ratio"; coeffCdCorrPR "Coefficient for discharge coefficient for pressure ratio"
  dmEmb_u : Outport
  dmEmb_d : Outport  Port=2
  aOpen : Outport  Port=3
  Cd : Outport  Port=4
  wires:
  S-Function/1 -> S-Function1/1  "ExhVVlift"
  IdealNozzleBus/2 -> dmEmb_d/1
  IdealNozzleBus/1 -> dmEmb_u/1
  phi/1 -> S-Function/1
  cAStartNom/1 -> S-Function/2
  dCALiftUp/1 -> S-Function/3
  S-Function1/3 -> IdealNozzleBus/1  "aEff"
  S-Function1/1 -> aOpen/1
  S-Function1/2 -> Cd/1
  pTF_u/1 -> IdealNozzleBus/2, Bus Selector/1
  Bus Selector/1 -> S-Function1/2  "<p>"
  pTF_d/1 -> IdealNozzleBus/3, Bus Selector1/1
  Bus Selector1/1 -> S-Function1/3  "<p>"

== system EngineSystemSubmodel/Components/ExhValveBusAEffAdjust ==
  phi : Inport
  cAStartNom : Inport  Port=2
  dCALiftUp : Inport  Port=3
  pTF_u : Inport  Port=4
  pTF_d : Inport  Port=5
  Bus Selector : BusSelector  OutputSignals=p
  Bus Selector1 : BusSelector  OutputSignals=p
  Constant : Constant  Value=cyl.exhVVDim.AEffFactor
  IdealNozzleBus : EngineSystemSubmodel/Flow Restriction/IdealNozzleBus
  Product : Product
  S-Function : S-Function  FunctionName=GetVVLift  Parameters=eng.nStroke,cyl.exhVVDim.liftMax,cyl.exhVVProf.cAStartRef,cyl.exhVVProf.dCALiftUp,cyl.exhVVProf.dCALiftDown,cyl.exhVVProf.dCALiftTopRef,cyl.exhVVProf.cAVVUpRef,cyl.exhVVProf.cAVVDownRef,cyl.exhVVProf.liftUpRef,cyl.exhVVProf.liftDownRef  EnableBusSupport=off
  S-Function1 : S-Function  FunctionName=GetExhVVArea  Parameters=cyl.exhVVDim.Dv,cyl.exhVVDim.beta,cyl.exhVVDim.w,cyl.exhVVDim.Dp,cyl.exhVVDim.Ds,coeffCdCorrP,coeffCdCorrQ,coeffCdCorrPR  EnableBusSupport=off  mask{coeffCdCorrP=[0.5329;-0.2047;0.04292], coeffCdCorrQ=[0.5359;-0.2962;0.06275], coeffCdCorrPR=[-0.006345;0.09503;0.8117]}
      mask prompts: coeffCdCorrP "Produt coefficient for discharge coefficient for lift ratio"; coeffCdCorrQ "Quotient coefficient for discharge coefficient for lift ratio"; coeffCdCorrPR "Coefficient for discharge coefficient for pressure ratio"
  dmEmb_u : Outport
  dmEmb_d : Outport  Port=2
  aOpen : Outport  Port=3
  Cd : Outport  Port=4
  wires:
  Bus Selector1/1 -> S-Function1/3  "<p>"
  pTF_d/1 -> Bus Selector1/1, IdealNozzleBus/3
  Bus Selector/1 -> S-Function1/2  "<p>"
  pTF_u/1 -> Bus Selector/1, IdealNozzleBus/2
  S-Function1/2 -> Cd/1
  S-Function1/1 -> aOpen/1
  dCALiftUp/1 -> S-Function/3
  cAStartNom/1 -> S-Function/2
  phi/1 -> S-Function/1
  IdealNozzleBus/1 -> dmEmb_u/1
  IdealNozzleBus/2 -> dmEmb_d/1
  S-Function/1 -> S-Function1/1  "ExhVVlift"
  Constant/1 -> Product/2
  S-Function1/3 -> Product/1  "aEff"
  Product/1 -> IdealNozzleBus/1

== system EngineSystemSubmodel/Components/InCylinderMV ==
  PTFu : Inport
  PTFd : Inport  Port=2
  omegae : Inport  Port=3
  throttle : Inport  Port=4
  Demux : Demux  Outputs=3
  Demux1 : Demux  Outputs=3
  Mux : Mux  Inputs=3
  Mux1 : Mux  Inputs=3
  S-Function : S-Function  FunctionName=InCylinderMV  Parameters=fs,Vd,LHV,Pe_nom,SFC,vol_eff_coeff1,vol_eff_coeff2,T_pe,nstroke,m_f_cyc_max,C1,p_a_inf,Pe0  SFunctionModules='GetThdynCombGasZach'  EnableBusSupport=off  mask{fs=fs, Vd=Vd, LHV=LHV, Pe_nom=Pe_nom, SFC=SFC, vol_eff_coeff1=vol_eff_coeff1, vol_eff_coeff2=vol_eff_coeff2, T_pe=T_pe, nstroke=nstroke, m_f_cyc_max=m_f_cyc_max, C1=C1, p_a_inf=p_a_inf, Pe0=Pe0}
      mask prompts: fs "Stoichiometric fuel air ratio"; Vd "Displacement volume [m3]"; LHV "Low heating value of the fuel [J/kg]"; Pe_nom "Rated power [W]"; SFC "Coefficient for the SFC model"; vol_eff_coeff1 "Coefficient for volumetric efficiency model for higher pressure"; vol_eff_coeff2 "Coefficient for volumetric efficiency model for lower pressure"; T_pe "Time constant for power development (0.01)"; nstroke "Number of stroke"; m_f_cyc_max "Maximum injected fuel per cycle"; C1 "Cofficient of heat transfer"; p_a_inf "Upper pressure limit for vol. eff. model change"; Pe0 "Initial power load"
  dmEmbu : Outport
  dmEmbd : Outport  Port=2
  Tqe : Outport  Port=3
  vol_eff : Outport  Port=4
  pe_pu : Outport  Port=5
  wires:
  S-Function/8 -> vol_eff/1
  S-Function/7 -> Tqe/1
  Mux1/1 -> dmEmbd/1
  S-Function/6 -> Mux1/3
  S-Function/5 -> Mux1/2
  S-Function/4 -> Mux1/1
  Mux/1 -> dmEmbu/1
  S-Function/3 -> Mux/3
  S-Function/2 -> Mux/2
  S-Function/1 -> Mux/1
  throttle/1 -> S-Function/8
  omegae/1 -> S-Function/7
  Demux1/3 -> S-Function/6
  Demux1/2 -> S-Function/5
  Demux1/1 -> S-Function/4
  PTFd/1 -> Demux1/1
  Demux/3 -> S-Function/3
  Demux/2 -> S-Function/2
  Demux/1 -> S-Function/1
  PTFu/1 -> Demux/1
  S-Function/9 -> pe_pu/1

== system EngineSystemSubmodel/Components/InCylinderMVBus ==
  pTFu : Inport
  pTFd : Inport  Port=2
  omegae : Inport  Port=3
  throttle : Inport  Port=4
  Bus Creator : BusCreator  Inputs=3
  Bus Creator1 : BusCreator  Inputs=3
  Bus Selector : BusSelector  OutputSignals=p,T,F
  Bus Selector1 : BusSelector  OutputSignals=p,T,F
  S-Function : S-Function  FunctionName=InCylinderMV  Parameters=eng.fs,cyl.dim.vD*eng.nCyl,eng.hn,eng.powNom,eng.SFC,cyl.volEffCoeff1,cyl.volEffCoeff2,cyl.tPe,eng.nStroke,cyl.comb.mqfCycMax*eng.nCyl,cyl.HT.C1,cyl.pAInf,cyl.Pe0  SFunctionModules=m  EnableBusSupport=off
  dmEmbu : Outport
  dmEmbd : Outport  Port=2
  Tqe : Outport  Port=3
  vol_eff : Outport  Port=4
  pe_pu : Outport  Port=5
  wires:
  S-Function/8 -> vol_eff/1  "volEff"
  S-Function/7 -> Tqe/1
  Bus Creator1/1 -> dmEmbd/1
  Bus Creator/1 -> dmEmbu/1
  S-Function/3 -> Bus Creator/3  "dmbu"
  S-Function/2 -> Bus Creator/2  "dEu"
  S-Function/1 -> Bus Creator/1  "dmu"
  throttle/1 -> S-Function/8
  omegae/1 -> S-Function/7
  S-Function/9 -> pe_pu/1
  S-Function/4 -> Bus Creator1/1  "dmd"
  S-Function/6 -> Bus Creator1/3  "dmbd"
  S-Function/5 -> Bus Creator1/2  "dEd"
  pTFu/1 -> Bus Selector/1
  pTFd/1 -> Bus Selector1/1
  Bus Selector/2 -> S-Function/2  "<T>"
  Bus Selector/1 -> S-Function/1  "<p>"
  Bus Selector/3 -> S-Function/3  "<F>"
  Bus Selector1/2 -> S-Function/5  "<T>"
  Bus Selector1/1 -> S-Function/4  "<p>"
  Bus Selector1/3 -> S-Function/6  "<F>"

== system EngineSystemSubmodel/Components/IntakePort ==
  phi : Inport
  pTF_u : Inport  Port=2
  pTF_d : Inport  Port=3
  IdealNozzle : EngineSystemSubmodel/Flow Restriction/IdealNozzle
  S-Function : S-Function  FunctionName=GetInportArea  Parameters=eng.nStroke,cyl.dim.S/2,cyl.dim.lambda,cyl.scavPort.X,cyl.scavPort.Y,cyl.scavPort.r,cyl.scavPort.nPort,cyl.dim.S  EnableBusSupport=off
  dmEmb_u : Outport
  dmEmb_d : Outport  Port=2
  aOpen : Outport  Port=3
  Cd : Outport  Port=4
  xP : Outport  Port=5
  wires:
  S-Function/2 -> Cd/1
  S-Function/1 -> aOpen/1
  pTF_d/1 -> IdealNozzle/3
  pTF_u/1 -> IdealNozzle/2
  IdealNozzle/2 -> dmEmb_d/1
  IdealNozzle/1 -> dmEmb_u/1
  phi/1 -> S-Function/1
  S-Function/3 -> IdealNozzle/1  "aEff"
  S-Function/4 -> xP/1

== system EngineSystemSubmodel/Components/IntakePortBus ==
  phi : Inport
  pTF_u : Inport  Port=2
  pTF_d : Inport  Port=3
  IdealNozzleBus : EngineSystemSubmodel/Flow Restriction/IdealNozzleBus
  S-Function : S-Function  FunctionName=GetInportArea  Parameters=eng.nStroke,cyl.dim.S/2,cyl.dim.lambda,cyl.scavPort.X,cyl.scavPort.Y,cyl.scavPort.r,cyl.scavPort.nPort,cyl.dim.S  EnableBusSupport=off
  dmEmb_u : Outport
  dmEmb_d : Outport  Port=2
  aOpen : Outport  Port=3
  Cd : Outport  Port=4
  xP : Outport  Port=5
  wires:
  S-Function/2 -> Cd/1
  S-Function/1 -> aOpen/1
  pTF_d/1 -> IdealNozzleBus/3
  pTF_u/1 -> IdealNozzleBus/2
  IdealNozzleBus/2 -> dmEmb_d/1
  IdealNozzleBus/1 -> dmEmb_u/1
  phi/1 -> S-Function/1
  S-Function/3 -> IdealNozzleBus/1  "aEff"
  S-Function/4 -> xP/1

== system EngineSystemSubmodel/Components/IntakeValve ==
  phi : Inport
  cAStartNom : Inport  Port=2
  dCALiftUp : Inport  Port=3
  pTF_u : Inport  Port=4
  pTF_d : Inport  Port=5
  Demux : Demux  Outputs=3
  Demux1 : Demux  Outputs=3
  IdealNozzle : EngineSystemSubmodel/Flow Restriction/IdealNozzle
  S-Function : S-Function  FunctionName=GetVVLift  Parameters=eng.nStroke,cyl.intakeVVDim.liftMax,cyl.intakeVVProf.cAStartRef,cyl.intakeVVProf.dCALiftUp,cyl.intakeVVProf.dCALiftDown,cyl.intakeVVProf.dCALiftTopRef,cyl.intakeVVProf.cAVVUpRef,cyl.intakeVVProf.cAVVDownRef,cyl.intakeVVProf.liftUpRef,cyl.intakeVVProf.liftDownRef  EnableBusSupport=off
  S-Function1 : S-Function  FunctionName=GetIntakeVVArea  Parameters=cyl.intakeVVDim.Dv,cyl.intakeVVDim.beta,cyl.intakeVVDim.w,cyl.intakeVVDim.Dp,cyl.intakeVVDim.Ds  EnableBusSupport=off
  Terminator{,1..3} (4 alike) : Terminator
  dmEmb_u : Outport
  dmEmb_d : Outport  Port=2
  aOpen : Outport  Port=3
  Cd : Outport  Port=4
  wires:
  Demux1/3 -> Terminator3/1
  Demux1/2 -> Terminator2/1
  Demux/3 -> Terminator1/1
  Demux/2 -> Terminator/1
  Demux1/1 -> S-Function1/3  "pOut"
  Demux/1 -> S-Function1/2  "pIn"
  S-Function1/2 -> Cd/1
  S-Function1/1 -> aOpen/1
  S-Function1/3 -> IdealNozzle/1  "aEff"
  dCALiftUp/1 -> S-Function/3
  cAStartNom/1 -> S-Function/2
  phi/1 -> S-Function/1
  IdealNozzle/1 -> dmEmb_u/1
  IdealNozzle/2 -> dmEmb_d/1
  pTF_u/1 -> IdealNozzle/2, Demux/1
  pTF_d/1 -> IdealNozzle/3, Demux1/1
  S-Function/1 -> S-Function1/1  "intakeVVlift"

== system EngineSystemSubmodel/Components/IntakeValveBus ==
  phi : Inport
  cAStartNom : Inport  Port=2
  dCALiftUp : Inport  Port=3
  pTF_u : Inport  Port=4
  pTF_d : Inport  Port=5
  Bus Selector : BusSelector  OutputSignals=p
  Bus Selector1 : BusSelector  OutputSignals=p
  IdealNozzleBus : EngineSystemSubmodel/Flow Restriction/IdealNozzleBus
  S-Function : S-Function  FunctionName=GetVVLift  Parameters=eng.nStroke,cyl.intakeVVDim.liftMax,cyl.intakeVVProf.cAStartRef,cyl.intakeVVProf.dCALiftUp,cyl.intakeVVProf.dCALiftDown,cyl.intakeVVProf.dCALiftTopRef,cyl.intakeVVProf.cAVVUpRef,cyl.intakeVVProf.cAVVDownRef,cyl.intakeVVProf.liftUpRef,cyl.intakeVVProf.liftDownRef  EnableBusSupport=off
  S-Function1 : S-Function  FunctionName=GetIntakeVVArea  Parameters=cyl.intakeVVDim.Dv,cyl.intakeVVDim.beta,cyl.intakeVVDim.w,cyl.intakeVVDim.Dp,cyl.intakeVVDim.Ds  EnableBusSupport=off
  dmEmb_u : Outport
  dmEmb_d : Outport  Port=2
  aOpen : Outport  Port=3
  Cd : Outport  Port=4
  wires:
  S-Function1/2 -> Cd/1
  S-Function1/1 -> aOpen/1
  S-Function1/3 -> IdealNozzleBus/1  "aEff"
  dCALiftUp/1 -> S-Function/3
  cAStartNom/1 -> S-Function/2
  phi/1 -> S-Function/1
  IdealNozzleBus/1 -> dmEmb_u/1
  IdealNozzleBus/2 -> dmEmb_d/1
  pTF_u/1 -> Bus Selector/1, IdealNozzleBus/2
  pTF_d/1 -> Bus Selector1/1, IdealNozzleBus/3
  S-Function/1 -> S-Function1/1  "intakeVVlift"
  Bus Selector/1 -> S-Function1/2  "<p>"
  Bus Selector1/1 -> S-Function1/3  "<p>"

== system EngineSystemSubmodel/Components/IntakeValveBusAEffAdjust ==
  phi : Inport
  cAStartNom : Inport  Port=2
  dCALiftUp : Inport  Port=3
  pTF_u : Inport  Port=4
  pTF_d : Inport  Port=5
  Bus Selector : BusSelector  OutputSignals=p
  Bus Selector1 : BusSelector  OutputSignals=p
  Constant : Constant  Value=cyl.intakeVVDim.AEffFactor
  IdealNozzleBus : EngineSystemSubmodel/Flow Restriction/IdealNozzleBus
  Product : Product
  S-Function : S-Function  FunctionName=GetVVLift  Parameters=eng.nStroke,cyl.intakeVVDim.liftMax,cyl.intakeVVProf.cAStartRef,cyl.intakeVVProf.dCALiftUp,cyl.intakeVVProf.dCALiftDown,cyl.intakeVVProf.dCALiftTopRef,cyl.intakeVVProf.cAVVUpRef,cyl.intakeVVProf.cAVVDownRef,cyl.intakeVVProf.liftUpRef,cyl.intakeVVProf.liftDownRef  EnableBusSupport=off
  S-Function1 : S-Function  FunctionName=GetIntakeVVArea  Parameters=cyl.intakeVVDim.Dv,cyl.intakeVVDim.beta,cyl.intakeVVDim.w,cyl.intakeVVDim.Dp,cyl.intakeVVDim.Ds  EnableBusSupport=off
  dmEmb_u : Outport
  dmEmb_d : Outport  Port=2
  aOpen : Outport  Port=3
  Cd : Outport  Port=4
  wires:
  Bus Selector1/1 -> S-Function1/3  "<p>"
  Bus Selector/1 -> S-Function1/2  "<p>"
  S-Function/1 -> S-Function1/1  "intakeVVlift"
  pTF_d/1 -> IdealNozzleBus/3, Bus Selector1/1
  pTF_u/1 -> IdealNozzleBus/2, Bus Selector/1
  IdealNozzleBus/2 -> dmEmb_d/1
  IdealNozzleBus/1 -> dmEmb_u/1
  phi/1 -> S-Function/1
  cAStartNom/1 -> S-Function/2
  dCALiftUp/1 -> S-Function/3
  S-Function1/3 -> Product/1  "aEff"
  S-Function1/1 -> aOpen/1
  S-Function1/2 -> Cd/1
  Constant/1 -> Product/2
  Product/1 -> IdealNozzleBus/1

== system EngineSystemSubmodel/Components/Turbocharger ==
  pTF_c_u : Inport
  pTF_c_d : Inport  Port=2
  pTF_t_u : Inport  Port=3
  pTF_t_d : Inport  Port=4
  Compressor1 : EngineSystemSubmodel/Flow Restriction/Compressor  comp=turbo.comp
  Constant : Constant  Value=turbo.jTC
  Integrator : Integrator  InitialCondition=turbo.omegaT0*turbo.jTC
  Product : Product  Inputs=*/
  Sum : Sum  Inputs=-|+
  Terminator : Terminator
  Terminator1 : Terminator
  Turbine1 : EngineSystemSubmodel/Flow Restriction/Turbine  turb=turbo.turb
  dmEmb_c_u : Outport
  dmEmb_c_d : Outport  Port=2
  dmEmb_t_u : Outport  Port=3
  dmEmb_t_d : Outport  Port=4
  T_t_d_calc : Outport  Port=5
  wires:
  pTF_c_d/1 -> Compressor1/2
  Turbine1/3 -> Sum/2  "tqTurb"
  Turbine1/1 -> dmEmb_t_u/1
  Compressor1/1 -> dmEmb_c_u/1
  Product/1 -> Turbine1/3, Compressor1/3  "omegat"
  Compressor1/2 -> dmEmb_c_d/1
  Integrator/1 -> Product/1
  Sum/1 -> Integrator/1
  Compressor1/3 -> Sum/1  "tqComp"
  Turbine1/2 -> dmEmb_t_d/1
  Turbine1/4 -> T_t_d_calc/1  "tempATurb"
  pTF_c_u/1 -> Compressor1/1
  pTF_t_u/1 -> Turbine1/1
  pTF_t_d/1 -> Turbine1/2
  Constant/1 -> Product/2
  Compressor1/4 -> Terminator/1  "effComp"
  Turbine1/5 -> Terminator1/1  "effTurb"
